simulink model "TryeSim"  (R2018a)
settings: Solver=FixedStepAuto  StartTime=0.0  StopTime=700  FixedStep=1  MaxStep=14.0  RelTol=1e-3
settings Model: Creator=sebastiankoch  LastModifiedBy=sebastiankoch
settings SolverCC: ZeroCrossAlgorithm=Adaptive
settings DebuggingCC: MaxConsecutiveZCsMsg=none

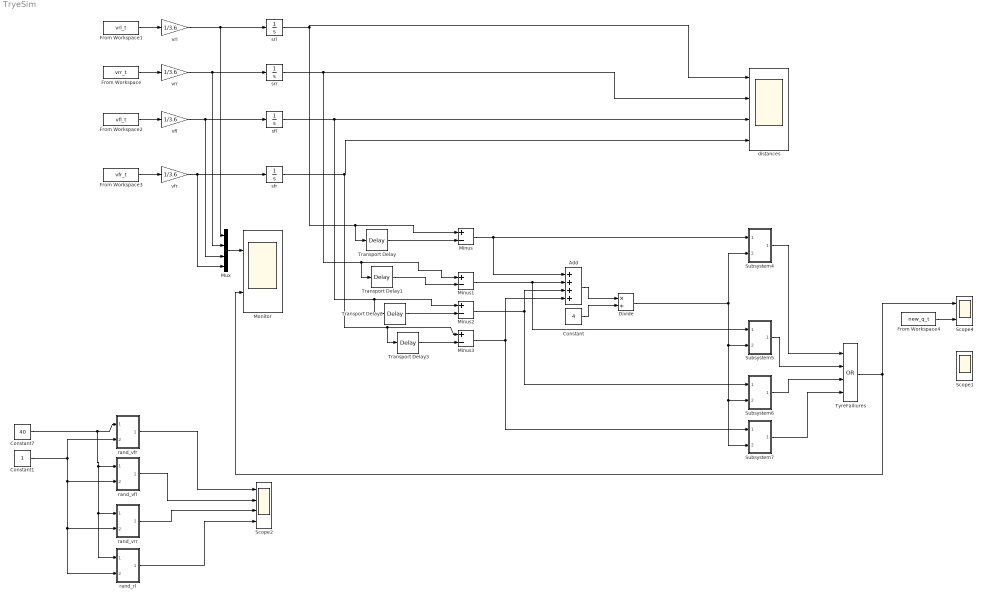
== system TryeSim ==
  Add : Sum  Inputs=4
  Constant : Constant  Value=4
  Constant1 : Constant
  Constant7 : Constant  Value=40
  Divide : Product  Inputs=*/
  From Workspace : FromWorkspace  VariableName=vrr_t  SampleTime=0
  From Workspace1 : FromWorkspace  VariableName=vrl_t  SampleTime=0
  From Workspace2 : FromWorkspace  VariableName=vfl_t  SampleTime=0
  From Workspace3 : FromWorkspace  VariableName=vfr_t  SampleTime=0
  From Workspace4 : FromWorkspace  VariableName=new_q_t
  Minus{,1..3} (4 alike) : Sum  Inputs=+-
  Monitor : Scope  NumInputPorts=2
  Mux : Mux
  Scope1 : Scope  NumInputPorts=2
  Scope2 : Scope  NumInputPorts=4
  Scope4 : Scope  NumInputPorts=2
  Subsystem4 : Subsystem
  Subsystem5 : Subsystem
  Subsystem6 : Subsystem
  Subsystem7 : Subsystem
  Transport Delay{,1..3} (4 alike) : TransportDelay
  TyreFailiures : Logic  Operator=OR  Inputs=4  AllPortsSameDT=off  OutDataTypeStr=boolean
  distances : Scope  NumInputPorts=4
  rand_rl : Subsystem
  rand_vfl : Subsystem
  rand_vfr : Subsystem
  rand_vrr : Subsystem
  sfl : Integrator
  sfr : Integrator
  srl : Integrator
  srr : Integrator
  vfl : Gain  Gain=1/3.6
  vfr : Gain  Gain=1/3.6
  vrl : Gain  Gain=1/3.6
  vrr : Gain  Gain=1/3.6
  wires:
  srl/1 -> distances/1, Minus/1, Transport Delay/1
  Constant/1 -> Divide/2
  Add/1 -> Divide/1
  From Workspace1/1 -> vrl/1
  From Workspace/1 -> vrr/1
  From Workspace2/1 -> vfl/1
  From Workspace3/1 -> vfr/1
  Transport Delay/1 -> Minus/2
  Transport Delay1/1 -> Minus1/2
  srr/1 -> Minus1/1, Transport Delay1/1, distances/2
  sfl/1 -> Minus2/1, Transport Delay2/1, distances/3
  Transport Delay2/1 -> Minus2/2
  sfr/1 -> Minus3/1, Transport Delay3/1, distances/4
  Transport Delay3/1 -> Minus3/2
  Minus1/1 -> Subsystem5/1(In1), Add/2
  Minus2/1 -> Subsystem6/1(In1), Add/3
  Minus3/1 -> Subsystem7/1(In1), Add/4
  From Workspace4/1 -> Scope4/2
  Subsystem4/1(Out1) -> TyreFailiures/1
  Subsystem5/1(Out1) -> TyreFailiures/2
  Subsystem6/1(Out1) -> TyreFailiures/3
  Subsystem7/1(Out1) -> TyreFailiures/4
  Minus/1 -> Add/1, Subsystem4/1(In1)
  Divide/1 -> Subsystem5/2(In2), Subsystem6/2(In2), Subsystem7/2(In2), Subsystem4/2(In2)
  Constant7/1 -> rand_vfl/1(In1), rand_rl/1(In1), rand_vrr/1(In1), rand_vfr/1(In1)
  rand_vfr/1(Out1) -> Scope2/1
  rand_vfl/1(Out1) -> Scope2/2
  rand_vrr/1(Out1) -> Scope2/3
  rand_rl/1(Out1) -> Scope2/4
  vrl/1 -> Mux/1, srl/1
  vrr/1 -> Mux/2, srr/1
  vfl/1 -> Mux/3, sfl/1
  vfr/1 -> Mux/4, sfr/1
  TyreFailiures/1 -> Monitor/2, Scope4/1
  Mux/1 -> Monitor/1
  ? -> Scope1/1
  Constant1/1 -> rand_rl/2(In2), rand_vrr/2(In2), rand_vfl/2(In2), rand_vfr/2(In2)

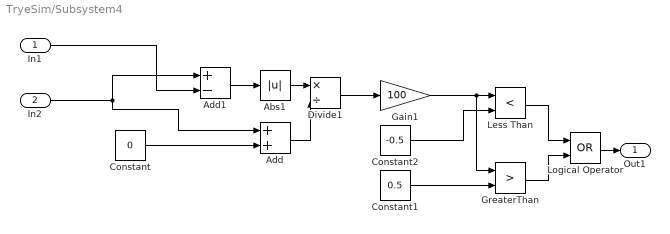
== system TryeSim/Subsystem4 ==
  In1 : Inport
  In2 : Inport  Port=2
  Abs1 : Abs
  Add : Sum
  Add1 : Sum  Inputs=+-
  Constant : Constant  Value=0
  Constant1 : Constant  Value=0.5
  Constant2 : Constant  Value=-0.5
  Divide1 : Product  Inputs=*/
  Gain1 : Gain  Gain=100
  GreaterThan : RelationalOperator  Operator=>  OutDataTypeStr=boolean  RndMeth=Simplest
  Less Than : RelationalOperator  Operator=<  OutDataTypeStr=boolean  RndMeth=Simplest
  Logical Operator : Logic  Operator=OR  AllPortsSameDT=off  OutDataTypeStr=boolean
  Out1 : Outport
  wires:
  Constant1/1 -> GreaterThan/2
  Less Than/1 -> Logical Operator/1
  GreaterThan/1 -> Logical Operator/2
  Constant2/1 -> Less Than/2
  Divide1/1 -> Gain1/1
  Logical Operator/1 -> Out1/1
  Gain1/1 -> GreaterThan/1, Less Than/1
  Constant/1 -> Add/2
  Add/1 -> Divide1/2
  In2/1 -> Add1/1, Add/1
  In1/1 -> Add1/2
  Add1/1 -> Abs1/1
  Abs1/1 -> Divide1/1

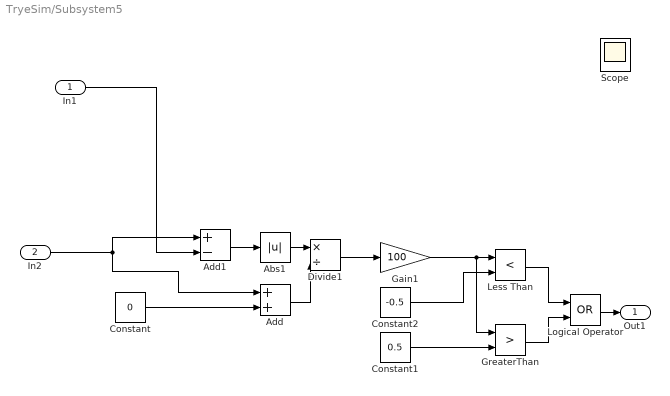
== system TryeSim/Subsystem5 ==
  In1 : Inport
  In2 : Inport  Port=2
  Abs1 : Abs
  Add : Sum
  Add1 : Sum  Inputs=+-
  Constant : Constant  Value=0
  Constant1 : Constant  Value=0.5
  Constant2 : Constant  Value=-0.5
  Divide1 : Product  Inputs=*/
  Gain1 : Gain  Gain=100
  GreaterThan : RelationalOperator  Operator=>  OutDataTypeStr=boolean  RndMeth=Simplest
  Less Than : RelationalOperator  Operator=<  OutDataTypeStr=boolean  RndMeth=Simplest
  Logical Operator : Logic  Operator=OR  AllPortsSameDT=off  OutDataTypeStr=boolean
  Scope : Scope  NumInputPorts=2
  Out1 : Outport
  wires:
  Abs1/1 -> Divide1/1
  Add1/1 -> Abs1/1
  In1/1 -> Add1/2
  In2/1 -> Add1/1, Add/1
  Add/1 -> Divide1/2
  Constant/1 -> Add/2
  Gain1/1 -> Less Than/1, GreaterThan/1
  Logical Operator/1 -> Out1/1
  Divide1/1 -> Gain1/1
  Constant2/1 -> Less Than/2
  GreaterThan/1 -> Logical Operator/2
  Less Than/1 -> Logical Operator/1
  Constant1/1 -> GreaterThan/2

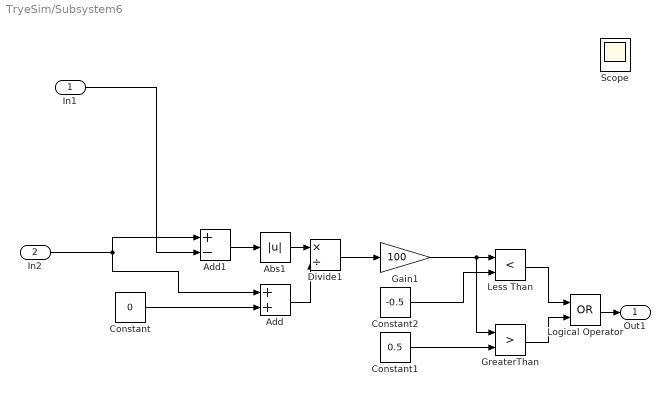
== system TryeSim/Subsystem6 ==
  In1 : Inport
  In2 : Inport  Port=2
  Abs1 : Abs
  Add : Sum
  Add1 : Sum  Inputs=+-
  Constant : Constant  Value=0
  Constant1 : Constant  Value=0.5
  Constant2 : Constant  Value=-0.5
  Divide1 : Product  Inputs=*/
  Gain1 : Gain  Gain=100
  GreaterThan : RelationalOperator  Operator=>  OutDataTypeStr=boolean  RndMeth=Simplest
  Less Than : RelationalOperator  Operator=<  OutDataTypeStr=boolean  RndMeth=Simplest
  Logical Operator : Logic  Operator=OR  AllPortsSameDT=off  OutDataTypeStr=boolean
  Scope : Scope  NumInputPorts=2
  Out1 : Outport
  wires:
  Constant1/1 -> GreaterThan/2
  Less Than/1 -> Logical Operator/1
  GreaterThan/1 -> Logical Operator/2
  Constant2/1 -> Less Than/2
  Divide1/1 -> Gain1/1
  Logical Operator/1 -> Out1/1
  Gain1/1 -> GreaterThan/1, Less Than/1
  Constant/1 -> Add/2
  Add/1 -> Divide1/2
  In2/1 -> Add/1, Add1/1
  In1/1 -> Add1/2
  Add1/1 -> Abs1/1
  Abs1/1 -> Divide1/1

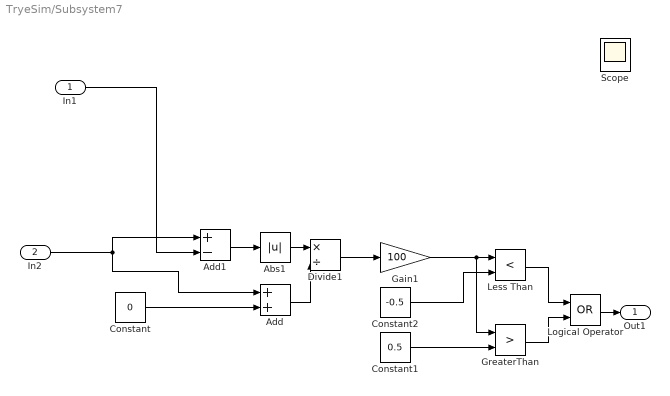
== system TryeSim/Subsystem7 ==
  In1 : Inport
  In2 : Inport  Port=2
  Abs1 : Abs
  Add : Sum
  Add1 : Sum  Inputs=+-
  Constant : Constant  Value=0
  Constant1 : Constant  Value=0.5
  Constant2 : Constant  Value=-0.5
  Divide1 : Product  Inputs=*/
  Gain1 : Gain  Gain=100
  GreaterThan : RelationalOperator  Operator=>  OutDataTypeStr=boolean  RndMeth=Simplest
  Less Than : RelationalOperator  Operator=<  OutDataTypeStr=boolean  RndMeth=Simplest
  Logical Operator : Logic  Operator=OR  AllPortsSameDT=off  OutDataTypeStr=boolean
  Scope : Scope  NumInputPorts=2
  Out1 : Outport
  wires:
  Abs1/1 -> Divide1/1
  Add1/1 -> Abs1/1
  In1/1 -> Add1/2
  In2/1 -> Add1/1, Add/1
  Add/1 -> Divide1/2
  Constant/1 -> Add/2
  Gain1/1 -> Less Than/1, GreaterThan/1
  Logical Operator/1 -> Out1/1
  Divide1/1 -> Gain1/1
  Constant2/1 -> Less Than/2
  GreaterThan/1 -> Logical Operator/2
  Less Than/1 -> Logical Operator/1
  Constant1/1 -> GreaterThan/2

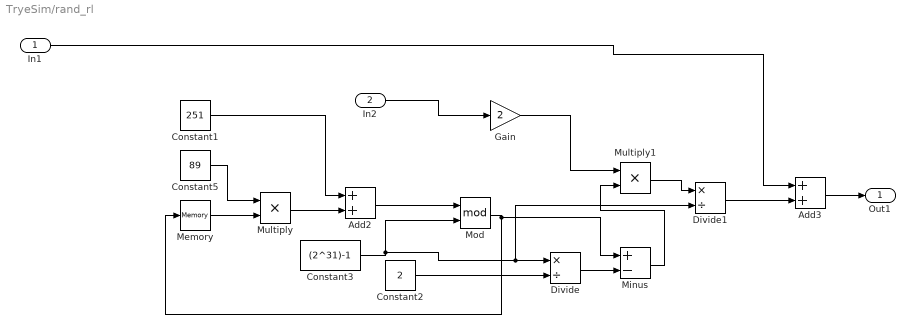
== system TryeSim/rand_rl ==
  In1 : Inport
  In2 : Inport  Port=2
  Add2 : Sum
  Add3 : Sum
  Constant1 : Constant  Value=251
  Constant2 : Constant  Value=2
  Constant3 : Constant  Value=(2^31)-1
  Constant5 : Constant  Value=89
  Divide : Product  Inputs=*/
  Divide1 : Product  Inputs=*/
  Gain : Gain  Gain=2
  Memory : Memory  InitialCondition=68676969868767687
  Minus : Sum  Inputs=+-
  Mod : Math  Operator=mod  SaturateOnIntegerOverflow=on
  Multiply : Product
  Multiply1 : Product
  Out1 : Outport
  wires:
  Constant2/1 -> Divide/2
  Divide/1 -> Minus/2
  Divide1/1 -> Add3/2
  Constant1/1 -> Add2/1
  Mod/1 -> Memory/1, Minus/1
  Multiply/1 -> Add2/2
  Memory/1 -> Multiply/2
  Add2/1 -> Mod/1
  Constant5/1 -> Multiply/1
  Add3/1 -> Out1/1
  Constant3/1 -> Mod/2, Divide1/2, Divide/1
  In1/1 -> Add3/1
  Minus/1 -> Multiply1/2
  Multiply1/1 -> Divide1/1
  Gain/1 -> Multiply1/1
  In2/1 -> Gain/1

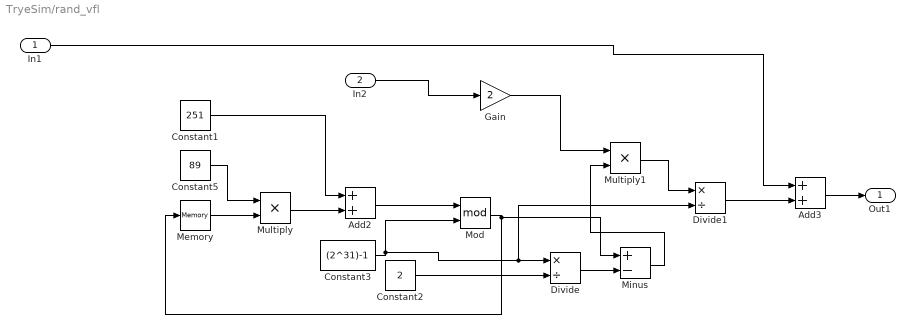
== system TryeSim/rand_vfl ==
  In1 : Inport
  In2 : Inport  Port=2
  Add2 : Sum
  Add3 : Sum
  Constant1 : Constant  Value=251
  Constant2 : Constant  Value=2
  Constant3 : Constant  Value=(2^31)-1
  Constant5 : Constant  Value=89
  Divide : Product  Inputs=*/
  Divide1 : Product  Inputs=*/
  Gain : Gain  Gain=2
  Memory : Memory  InitialCondition=780979809
  Minus : Sum  Inputs=+-
  Mod : Math  Operator=mod  SaturateOnIntegerOverflow=on
  Multiply : Product
  Multiply1 : Product
  Out1 : Outport
  wires:
  Constant2/1 -> Divide/2
  Divide/1 -> Minus/2
  Divide1/1 -> Add3/2
  Constant1/1 -> Add2/1
  Mod/1 -> Memory/1, Minus/1
  Multiply/1 -> Add2/2
  Memory/1 -> Multiply/2
  Add2/1 -> Mod/1
  Constant5/1 -> Multiply/1
  Add3/1 -> Out1/1
  Constant3/1 -> Mod/2, Divide1/2, Divide/1
  In1/1 -> Add3/1
  In2/1 -> Gain/1
  Gain/1 -> Multiply1/1
  Minus/1 -> Multiply1/2
  Multiply1/1 -> Divide1/1

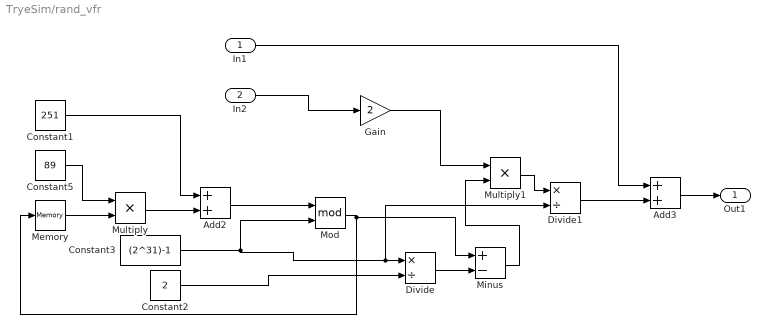
== system TryeSim/rand_vfr ==
  In1 : Inport
  In2 : Inport  Port=2
  Add2 : Sum
  Add3 : Sum
  Constant1 : Constant  Value=251
  Constant2 : Constant  Value=2
  Constant3 : Constant  Value=(2^31)-1
  Constant5 : Constant  Value=89
  Divide : Product  Inputs=*/
  Divide1 : Product  Inputs=*/
  Gain : Gain  Gain=2
  Memory : Memory  InitialCondition=7687676
  Minus : Sum  Inputs=+-
  Mod : Math  Operator=mod  SaturateOnIntegerOverflow=on
  Multiply : Product
  Multiply1 : Product
  Out1 : Outport
  wires:
  In1/1 -> Add3/1
  Constant3/1 -> Divide1/2, Divide/1, Mod/2
  Add3/1 -> Out1/1
  Constant5/1 -> Multiply/1
  Add2/1 -> Mod/1
  Memory/1 -> Multiply/2
  Multiply/1 -> Add2/2
  Mod/1 -> Minus/1, Memory/1
  Constant1/1 -> Add2/1
  Divide1/1 -> Add3/2
  Divide/1 -> Minus/2
  Constant2/1 -> Divide/2
  Minus/1 -> Multiply1/2
  Multiply1/1 -> Divide1/1
  In2/1 -> Gain/1
  Gain/1 -> Multiply1/1

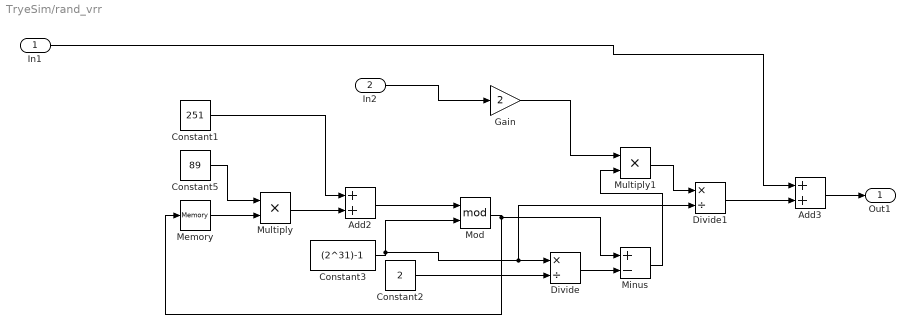
== system TryeSim/rand_vrr ==
  In1 : Inport
  In2 : Inport  Port=2
  Add2 : Sum
  Add3 : Sum
  Constant1 : Constant  Value=251
  Constant2 : Constant  Value=2
  Constant3 : Constant  Value=(2^31)-1
  Constant5 : Constant  Value=89
  Divide : Product  Inputs=*/
  Divide1 : Product  Inputs=*/
  Gain : Gain  Gain=2
  Memory : Memory  InitialCondition=3453
  Minus : Sum  Inputs=+-
  Mod : Math  Operator=mod  SaturateOnIntegerOverflow=on
  Multiply : Product
  Multiply1 : Product
  Out1 : Outport
  wires:
  In1/1 -> Add3/1
  Constant3/1 -> Divide1/2, Divide/1, Mod/2
  Add3/1 -> Out1/1
  Constant5/1 -> Multiply/1
  Add2/1 -> Mod/1
  Memory/1 -> Multiply/2
  Multiply/1 -> Add2/2
  Mod/1 -> Minus/1, Memory/1
  Constant1/1 -> Add2/1
  Divide1/1 -> Add3/2
  Divide/1 -> Minus/2
  Constant2/1 -> Divide/2
  Multiply1/1 -> Divide1/1
  Minus/1 -> Multiply1/2
  Gain/1 -> Multiply1/1
  In2/1 -> Gain/1
